simulink model "PAN_rendezvous_GNC_block_v3"  (R2017b)
settings: Solver=VariableStepAuto  StartTime=0.0  StopTime=10.0  RelTol=1e-3
values from neighbouring files (symbols this model uses):
  d_target = 2000    [variable_setup_v3.m]
  Imp_max = Imp_range(2)    [variable_setup_v3.m]
  Imp_min = Imp_range(1)    [variable_setup_v3.m]
  K_F = diag([1/norm(h0_t);1/norm(h0_t);1/norm(h0_t);1/abs(E0_t);1;1;1])    [variable_setup_v3.m]
  L_F = eye(3)    [variable_setup_v3.m]
  muE = 3.98600441500E+14    (= 398600441500000)    [variable_setup_v3.m]
  nsteps = 10000    [variable_setup_v3.m]
  nsteps_dr = 1000    [variable_setup_v3.m]
  rntol = 500    [variable_setup_v3.m]
  rtols = [500;500;50]    [variable_setup_v3.m]
libraries: hEemethod x7
settings Model: Creator=mtwal  LastModifiedBy=mtwal

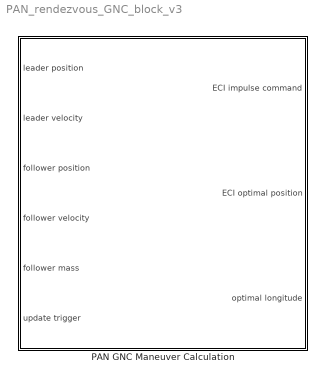
== system PAN_rendezvous_GNC_block_v3 ==
  PAN GNC Maneuver Calculation : Subsystem

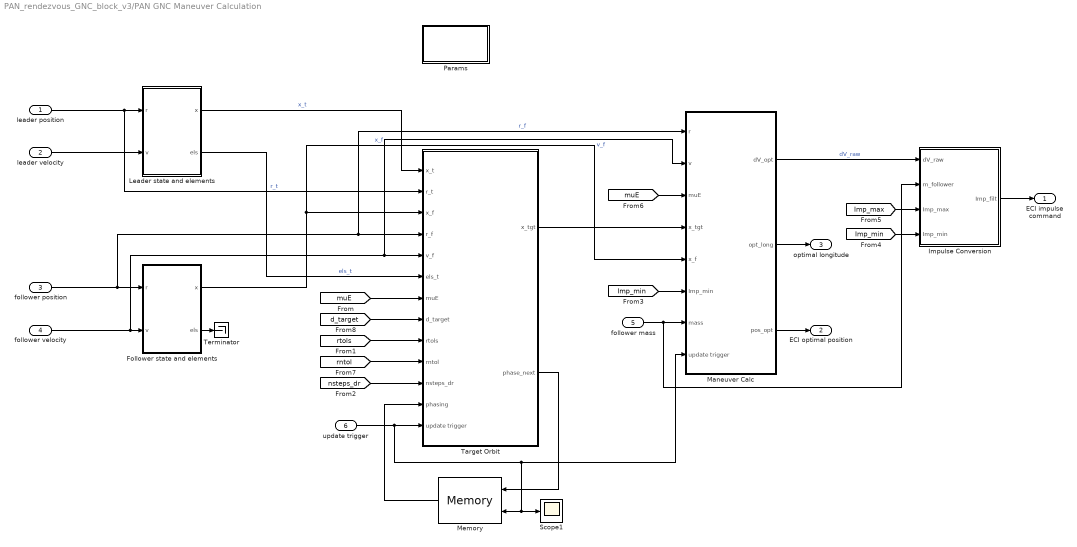
== system PAN_rendezvous_GNC_block_v3/PAN GNC Maneuver Calculation ==
  leader position : Inport
  leader velocity : Inport  Port=2
  follower position : Inport  Port=3
  follower velocity : Inport  Port=4
  follower mass : Inport  Port=5
  update trigger : Inport  Port=6
  Follower state and elements : Subsystem
  Impulse Conversion : MATLAB Function  TreatAsAtomicUnit=on
  Leader state and elements : Subsystem
  Maneuver Calc : Subsystem
  Memory : hEemethod/Simulation Blocks/Memory
      settings: SourceProductName=HEe Method Library
  Params : Subsystem
  Scope1 : Scope
  Target Orbit : Subsystem
  Terminator : Terminator
  ECI impulse command : Outport
  ECI optimal position : Outport  Port=2
  optimal longitude : Outport  Port=3
  wires:
  Impulse Conversion/1(Imp_filt) -> ECI impulse command/1
  [Imp_min] -> Maneuver Calc/6(Imp_min)
  [Imp_min] -> Impulse Conversion/4(Imp_min)
  [Imp_max] -> Impulse Conversion/3(Imp_max)
  leader position/1 -> Target Orbit/2(r_t), Leader state and elements/1(r)  "r_t"
  leader velocity/1 -> Leader state and elements/2(v)
  follower position/1 -> Maneuver Calc/1("r "), Target Orbit/4(r_f), Follower state and elements/1(r)  "r_f"
  follower velocity/1 -> Maneuver Calc/2("v "), Target Orbit/5(v_f), Follower state and elements/2(v)  "v_f"
  Follower state and elements/1(x) -> Target Orbit/3(x_f), Maneuver Calc/5(x_f)  "x_f"
  follower mass/1 -> Impulse Conversion/2(m_follower), Maneuver Calc/7(mass)
  Maneuver Calc/1(dV_opt) -> Impulse Conversion/1(dV_raw)  "dV_raw"
  [muE] -> Maneuver Calc/3(muE)
  Maneuver Calc/2(opt_long) -> optimal longitude/1
  Maneuver Calc/3(pos_opt) -> ECI optimal position/1
  Follower state and elements/2(els) -> Terminator/1
  update trigger/1 -> Maneuver Calc/8(update trigger), Scope1/1, Memory/2, Target Orbit/13(update trigger)
  Leader state and elements/1(x) -> Target Orbit/1(x_t)  "x_t"
  Leader state and elements/2(els) -> Target Orbit/6(els_t)  "els_t"
  [muE] -> Target Orbit/7(muE)
  [rtols] -> Target Orbit/9(rtols)
  [rntol] -> Target Orbit/10(rntol)
  [nsteps_dr] -> Target Orbit/11(nsteps_dr)
  Target Orbit/1(x_tgt) -> Maneuver Calc/4(x_tgt)
  Target Orbit/2(phase_next) -> Memory/1
  Memory/1 -> Target Orbit/12(phasing)
  [d_target] -> Target Orbit/8(d_target)

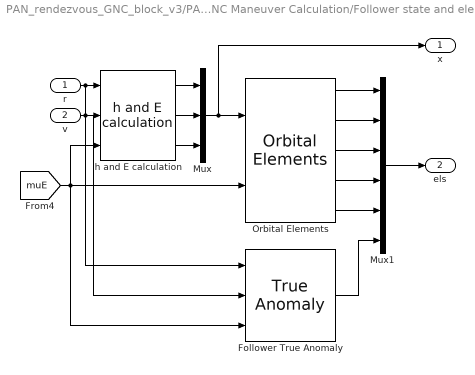
== system PAN_rendezvous_GNC_block_v3/PAN GNC Maneuver Calculation/Follower state and elements ==
  r : Inport
  v : Inport  Port=2
  Follower True Anomaly : hEemethod/Math Operations/True Anomaly
      settings: SourceProductName=HEe Method Library
  Mux : Mux  Inputs=3
  Mux1 : Mux  Inputs=6
  Orbital Elements : hEemethod/Math Operations/Orbital Elements
      settings: SourceProductName=HEe Method Library
  h and E calculation : hEemethod/Math Operations/h and E calculation
      settings: SourceProductName=HEe Method Library
  x : Outport
  els : Outport  Port=2
  wires:
  h and E calculation/1 -> Mux/1
  Orbital Elements/5 -> Mux1/5
  Orbital Elements/2 -> Mux1/2
  Orbital Elements/3 -> Mux1/3
  Orbital Elements/1 -> Mux1/1
  r/1 -> Follower True Anomaly/1, h and E calculation/1
  Orbital Elements/4 -> Mux1/4
  v/1 -> Follower True Anomaly/2, h and E calculation/2
  Mux/1 -> x/1, Orbital Elements/1
  h and E calculation/2 -> Mux/2
  h and E calculation/3 -> Mux/3
  [muE] -> Follower True Anomaly/3, Orbital Elements/2, h and E calculation/3
  Follower True Anomaly/1 -> Mux1/6
  Mux1/1 -> els/1

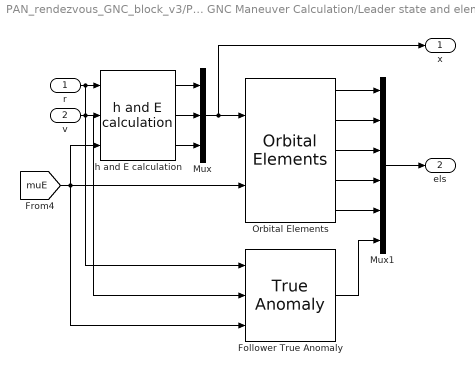
== system PAN_rendezvous_GNC_block_v3/PAN GNC Maneuver Calculation/Leader state and elements ==
  r : Inport
  v : Inport  Port=2
  Follower True Anomaly : hEemethod/Math Operations/True Anomaly
      settings: SourceProductName=HEe Method Library
  Mux : Mux  Inputs=3
  Mux1 : Mux  Inputs=6
  Orbital Elements : hEemethod/Math Operations/Orbital Elements
      settings: SourceProductName=HEe Method Library
  h and E calculation : hEemethod/Math Operations/h and E calculation
      settings: SourceProductName=HEe Method Library
  x : Outport
  els : Outport  Port=2
  wires:
  h and E calculation/1 -> Mux/1
  Orbital Elements/5 -> Mux1/5
  Orbital Elements/2 -> Mux1/2
  Orbital Elements/3 -> Mux1/3
  Orbital Elements/1 -> Mux1/1
  r/1 -> Follower True Anomaly/1, h and E calculation/1
  Orbital Elements/4 -> Mux1/4
  v/1 -> Follower True Anomaly/2, h and E calculation/2
  Mux/1 -> x/1, Orbital Elements/1
  h and E calculation/2 -> Mux/2
  h and E calculation/3 -> Mux/3
  [muE] -> Follower True Anomaly/3, Orbital Elements/2, h and E calculation/3
  Follower True Anomaly/1 -> Mux1/6
  Mux1/1 -> els/1

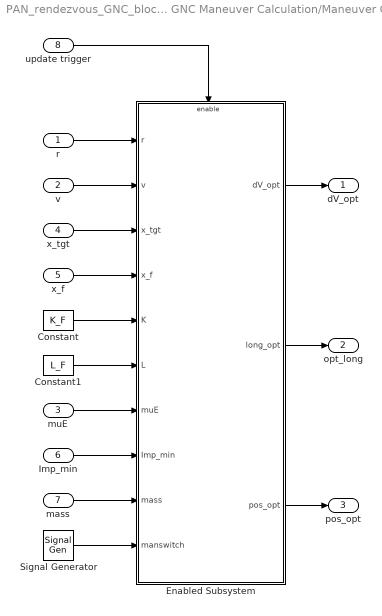
== system PAN_rendezvous_GNC_block_v3/PAN GNC Maneuver Calculation/Maneuver Calc ==
  "r " : Inport
  "v " : Inport  Port=2
  muE : Inport  Port=3
  x_tgt : Inport  Port=4
  x_f : Inport  Port=5
  Imp_min : Inport  Port=6
  mass : Inport  Port=7
  update trigger : Inport  Port=8
  Constant : Constant  Value=K_F
  Constant1 : Constant  Value=L_F
  Enabled Subsystem : Subsystem  TreatAsAtomicUnit=on
  Signal Generator : SignalGenerator  WaveForm=square  Frequency=2*pi/(2*5500)  Units=rad/sec
  dV_opt : Outport
  opt_long : Outport  Port=2
  pos_opt : Outport  Port=3
  wires:
  Enabled Subsystem/2(long_opt) -> opt_long/1
  "r "/1 -> Enabled Subsystem/1(r)
  "v "/1 -> Enabled Subsystem/2(v)
  muE/1 -> Enabled Subsystem/7("muE ")
  x_tgt/1 -> Enabled Subsystem/3(x_tgt)
  x_f/1 -> Enabled Subsystem/4(x_f)
  Constant/1 -> Enabled Subsystem/5(K)
  Constant1/1 -> Enabled Subsystem/6(L)
  Enabled Subsystem/1(dV_opt) -> dV_opt/1
  Enabled Subsystem/3(pos_opt) -> pos_opt/1
  Imp_min/1 -> Enabled Subsystem/8(Imp_min)
  mass/1 -> Enabled Subsystem/9(mass)
  update trigger/1 -> Enabled Subsystem/Enable
  Signal Generator/1 -> Enabled Subsystem/10(manswitch)

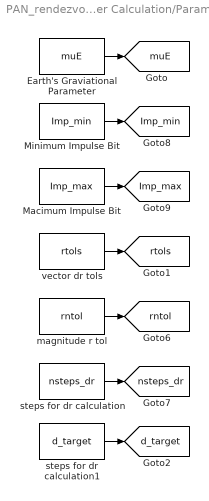
== system PAN_rendezvous_GNC_block_v3/PAN GNC Maneuver Calculation/Params ==
  Earth's Graviational Parameter : Constant  Value=muE
  Macimum Impulse Bit : Constant  Value=Imp_max
  Minimum Impulse Bit : Constant  Value=Imp_min
  magnitude r tol : Constant  Value=rntol
  steps for dr calculation : Constant  Value=nsteps_dr
  steps for dr calculation1 : Constant  Value=d_target
  vector dr tols : Constant  Value=rtols
  tag scope: Imp_max=global, Imp_min=global, d_target=global, muE=global, nsteps_dr=global, rntol=global, rtols=global
  wires:
  Earth's Graviational Parameter/1 -> [muE]
  Minimum Impulse Bit/1 -> [Imp_min]
  Macimum Impulse Bit/1 -> [Imp_max]
  magnitude r tol/1 -> [rntol]
  steps for dr calculation/1 -> [nsteps_dr]
  vector dr tols/1 -> [rtols]
  steps for dr calculation1/1 -> [d_target]

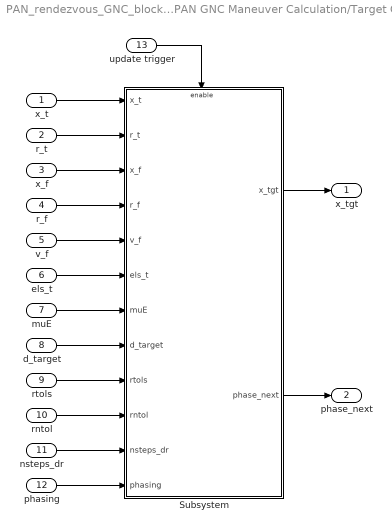
== system PAN_rendezvous_GNC_block_v3/PAN GNC Maneuver Calculation/Target Orbit ==
  x_t : Inport
  r_t : Inport  Port=2
  x_f : Inport  Port=3
  r_f : Inport  Port=4
  v_f : Inport  Port=5
  els_t : Inport  Port=6
  muE : Inport  Port=7
  d_target : Inport  Port=8
  rtols : Inport  Port=9
  rntol : Inport  Port=10
  nsteps_dr : Inport  Port=11
  phasing : Inport  Port=12
  update trigger : Inport  Port=13
  Subsystem : Subsystem
  x_tgt : Outport
  phase_next : Outport  Port=2
  wires:
  els_t/1 -> Subsystem/6(els_t)
  r_f/1 -> Subsystem/4(r_f)
  v_f/1 -> Subsystem/5(v_f)
  muE/1 -> Subsystem/7(muE)
  rtols/1 -> Subsystem/9(rtols)
  rntol/1 -> Subsystem/10(rntol)
  nsteps_dr/1 -> Subsystem/11(nsteps_dr)
  Subsystem/1(x_tgt) -> x_tgt/1
  Subsystem/2(phase_next) -> phase_next/1
  update trigger/1 -> Subsystem/Enable
  phasing/1 -> Subsystem/12(phasing)
  x_f/1 -> Subsystem/3(x_f)
  x_t/1 -> Subsystem/1(x_t)
  r_t/1 -> Subsystem/2(r_t)
  d_target/1 -> Subsystem/8(d_target)

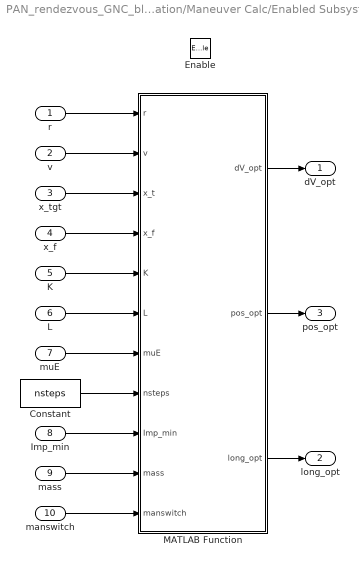
== system PAN_rendezvous_GNC_block_v3/PAN GNC Maneuver Calculation/Maneuver Calc/Enabled Subsystem ==
  r : Inport
  v : Inport  Port=2
  x_tgt : Inport  Port=3
  x_f : Inport  Port=4
  K : Inport  Port=5
  L : Inport  Port=6
  "muE " : Inport  Port=7
  Imp_min : Inport  Port=8
  mass : Inport  Port=9
  manswitch : Inport  Port=10
  Enable : EnablePort
  Constant : Constant  Value=nsteps
  MATLAB Function : MATLAB Function  TreatAsAtomicUnit=on
  dV_opt : Outport
  long_opt : Outport  Port=2
  pos_opt : Outport  Port=3
  wires:
  r/1 -> MATLAB Function/1(r)
  v/1 -> MATLAB Function/2(v)
  "muE "/1 -> MATLAB Function/7(muE)
  x_tgt/1 -> MATLAB Function/3(x_t)
  x_f/1 -> MATLAB Function/4(x_f)
  K/1 -> MATLAB Function/5(K)
  L/1 -> MATLAB Function/6(L)
  MATLAB Function/3(long_opt) -> long_opt/1
  MATLAB Function/1(dV_opt) -> dV_opt/1
  MATLAB Function/2(pos_opt) -> pos_opt/1
  Constant/1 -> MATLAB Function/8(nsteps)
  Imp_min/1 -> MATLAB Function/9(Imp_min)
  mass/1 -> MATLAB Function/10(mass)
  manswitch/1 -> MATLAB Function/11(manswitch)

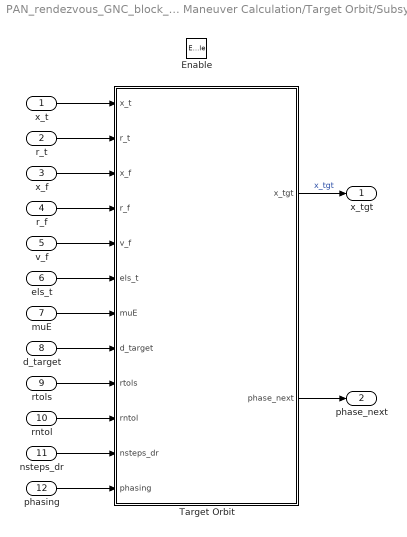
== system PAN_rendezvous_GNC_block_v3/PAN GNC Maneuver Calculation/Target Orbit/Subsystem ==
  x_t : Inport
  r_t : Inport  Port=2
  x_f : Inport  Port=3
  r_f : Inport  Port=4
  v_f : Inport  Port=5
  els_t : Inport  Port=6
  muE : Inport  Port=7
  d_target : Inport  Port=8
  rtols : Inport  Port=9
  rntol : Inport  Port=10
  nsteps_dr : Inport  Port=11
  phasing : Inport  Port=12
  Enable : EnablePort
  Target Orbit : MATLAB Function  TreatAsAtomicUnit=on
  x_tgt : Outport
  phase_next : Outport  Port=2
  wires:
  rntol/1 -> Target Orbit/10(rntol)
  v_f/1 -> Target Orbit/5(v_f)
  r_t/1 -> Target Orbit/2(r_t)
  Target Orbit/2(phase_next) -> phase_next/1
  r_f/1 -> Target Orbit/4(r_f)
  phasing/1 -> Target Orbit/12(phasing)
  muE/1 -> Target Orbit/7(muE)
  els_t/1 -> Target Orbit/6(els_t)
  Target Orbit/1(x_tgt) -> x_tgt/1  "x_tgt"
  nsteps_dr/1 -> Target Orbit/11(nsteps_dr)
  x_t/1 -> Target Orbit/1(x_t)
  rtols/1 -> Target Orbit/9(rtols)
  x_f/1 -> Target Orbit/3(x_f)
  d_target/1 -> Target Orbit/8(d_target)

== matlab function PAN_rendezvous_GNC_block_v3/PAN GNC Maneuver Calculation/Target Orbit/Subsystem/Target Orbit ==
  data: x_t input; r_t input; x_f input; r_f input; v_f input; els_t input; muE input; d_target input; rtols input; rntol input; x_tgt output; nsteps_dr input; phasing input; phase_next output
function [x_tgt,phase_next] = targetOrbit(x_t,r_t,x_f,r_f,v_f,els_t,muE,d_target,rtols,rntol,nsteps_dr,phasing)

pos_diff = r_t-r_f;
vhat = v_f/norm(v_f);
dr_vbar = dot(vhat,pos_diff)*vhat;
along_track_sep = norm(dr_vbar);
follower_ahead = (dot(vhat,pos_diff) < 0);
[matched,~] = orb_matched_dr(x_t,x_f,muE,nsteps_dr,rtols,rntol);

if (~matched && ~phasing)
    x_tgt = x_t;
    phase_next = 0;
elseif (norm(pos_diff) < d_target)
    x_tgt = x_t;
    phase_next = 0;
else
    if (norm(pos_diff) > 500000)
        if (follower_ahead)
            da_tgt = 50;
        else
            da_tgt = -50;
        end
    else
        [da_tgt,~] = decel_step_PAN(along_track_sep,follower_ahead);
    end

    a_tgt = els_t(1) + da_tgt;
    
%     if (norm(pos_diff) < d_target)
%         phase_next = 0;
%     else
        phase_next = 1;
%     end

    [~,~,x_tgt]=phasing_orbit(els_t,a_tgt,muE);
end

end

== matlab function PAN_rendezvous_GNC_block_v3/PAN GNC Maneuver Calculation/Maneuver Calc/Enabled Subsystem/MATLAB Function ==
  data: dV_opt output; pos_opt output; long_opt output; r input; v input; x_t input; x_f input; K input; L input; muE input; nsteps input; Imp_min input; mass input; manswitch input
function [dV_opt,pos_opt,long_opt] = fcn(r,v,x_t,x_f,K,L,muE,nsteps,Imp_min,mass,manswitch)
%#codegen

z0=[r;v];

E=norm(v)^2/2-muE/norm(r);
a=-muE/(2*E);
T=2*pi/sqrt(muE)*a^(3/2);

options=odeset('AbsTol',1e-12,'RelTol',1e-12);
tspan=linspace(0,T,nsteps);
[~,zs] = ode45(@kepler_diff,tspan,z0,options,muE,[0;0;0]);

dV_opt = [0;0;0];
pos_opt = [0;0;0];
long_opt = 0;
R_max = 0;
R_j = 0;
dx=x_t-x_f;

for i=1:nsteps
    r_j = zs(i,1:3);
    v_j = zs(i,4:6);
    h_j = cross(r_j,v_j);
    
    Mh = crs(r_j);
    ME = v_j;
    Me = (crs(v_j)*crs(r_j)-crs(h_j))/muE;
    
    if (manswitch)
        % angular momentum maneuver
        M = [Mh;ME;Me];
    else
        % eccentrcity maneuver
        M = [zeros(4,3);Me];
    end
    
    dV_j = pinv(M)*dx;
    dx_j = M*dV_j;

    if (norm(dV_j)*mass < norm(Imp_min))
        R_j=-999999;
    else
        dx_j_use = dot(dx_j,dx)/(norm(dx_j)*norm(dx))*dx;
        dx_j_opt_sqd = dx_j_use'*K*dx_j_use;
        dV_j_sqd = dV_j'*L*dV_j;
        R_j = dx_j_opt_sqd/dV_j_sqd;
    end

    if (R_j>R_max)
        R_max = R_j;
        long_opt = atan2(r_j(2),r_j(1));
        pos_opt = r_j';
        dV_opt = dV_j;
        if (long_opt<0)
            long_opt=long_opt+2*pi;
        end
    end
end

end

== matlab function PAN_rendezvous_GNC_block_v3/PAN GNC Maneuver Calculation/Impulse Conversion ==
  data: dV_raw input; m_follower input; Imp_filt output; Imp_max input; Imp_min input
function Imp_filt = fcn(dV_raw,m_follower,Imp_max,Imp_min)
%#codegen

Imp_raw = dV_raw*m_follower;

if (norm(Imp_raw)>Imp_max)
    Imp_red=Imp_raw*(Imp_max/norm(Imp_raw));
elseif (norm(Imp_raw)<Imp_min)
    Imp_red=[0;0;0];
else
    Imp_red=Imp_raw;
end

Imp_filt = Imp_red;
